simulink model "model_LQR"  (R2021b)
settings: Solver=VariableStepAuto  StartTime=0.0  StopTime=T  RelTol=1e-3
undefined symbols (not defined in the file): DiscIntNeverNeededParam
settings Model: Creator=mateusz  LastModifiedBy=mateusz

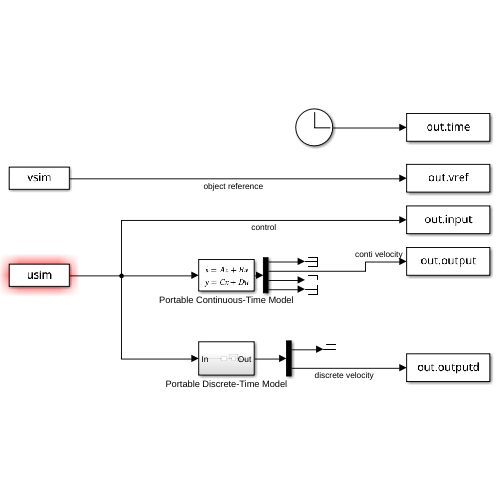
[thumbnail: Simulink's stored preview of the top-level diagram]
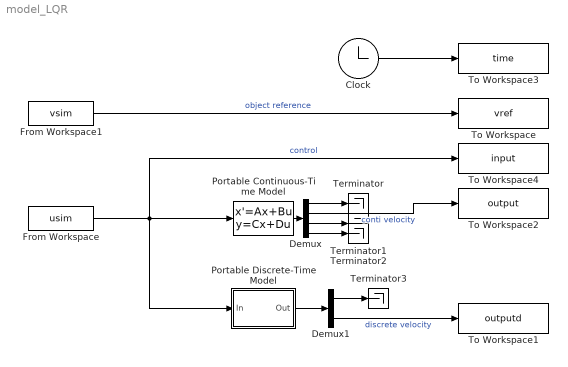
== system model_LQR ==
  Clock : Clock
  Demux : Demux
  Demux1 : Demux  Outputs=2
  From Workspace : FromWorkspace  VariableName=usim
  From Workspace1 : FromWorkspace  VariableName=vsim
  Portable Continuous-Time Model : StateSpace  A=|  B=[0;0;0;2.59e4];  C=eye(4,4)  D=zeros(4,1)  InitialCondition=0
      | [0  1  0    0;
      |      0 -5  4.5  0;
      |      0  0 -0.7108*2  23.6012*2;
      |      0  0 -5.3898 -4040];
  Portable Discrete-Time Model : Subsystem
  Terminator{,1..3} (4 alike) : Terminator
  To Workspace : ToWorkspace  VariableName=vref  SampleTime=0.02
  To Workspace1 : ToWorkspace  VariableName=outputd  SampleTime=0.02
  To Workspace2 : ToWorkspace  VariableName=output  SampleTime=0.02
  To Workspace3 : ToWorkspace  VariableName=time  SampleTime=0.02
  To Workspace4 : ToWorkspace  VariableName=input  SampleTime=0.02
  wires:
  Portable Continuous-Time Model/1 -> Demux/1
  From Workspace/1 -> To Workspace4/1, Portable Discrete-Time Model/1(In), Portable Continuous-Time Model/1  "control"
  Portable Discrete-Time Model/1(Out) -> Demux1/1
  From Workspace1/1 -> To Workspace/1  "object reference"
  Demux/1 -> Terminator/1
  Demux/3 -> Terminator1/1
  Demux/4 -> Terminator2/1
  Demux1/1 -> Terminator3/1
  Demux/2 -> To Workspace2/1  "conti velocity"
  Demux1/2 -> To Workspace1/1  "discrete velocity"
  Clock/1 -> To Workspace3/1

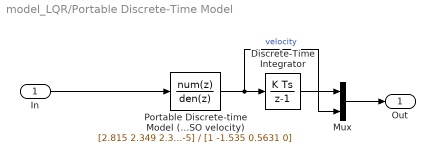
== system model_LQR/Portable Discrete-Time Model ==
  In : Inport
  Discrete-Time Integrator : DiscreteIntegrator  SampleTime=-1  ICPrevOutput=DiscIntNeverNeededParam  ICPrevScaledInput=DiscIntNeverNeededParam
  Mux : Mux  Inputs=2
  Portable Discrete-time Model (SISO velocity) : DiscreteTransferFcn  Numerator=[2.815 2.349 2.353e-5]  Denominator=[1 -1.535 0.5631 0]  SampleTime=0.1
  Out : Outport
  wires:
  In/1 -> Portable Discrete-time Model (SISO velocity)/1
  Portable Discrete-time Model (SISO velocity)/1 -> Mux/2, Discrete-Time Integrator/1  "velocity"
  Mux/1 -> Out/1
  Discrete-Time Integrator/1 -> Mux/1
